simulink model "lab2_part3"  (R2023a)
settings: Solver=ode45  StartTime=0.0  StopTime=3  RelTol=1e-3
undefined symbols (not defined in the file or in its folder): a, zeta
settings Model: Creator=Jiadong_Hong  LastModifiedBy=Jiadong_Hong

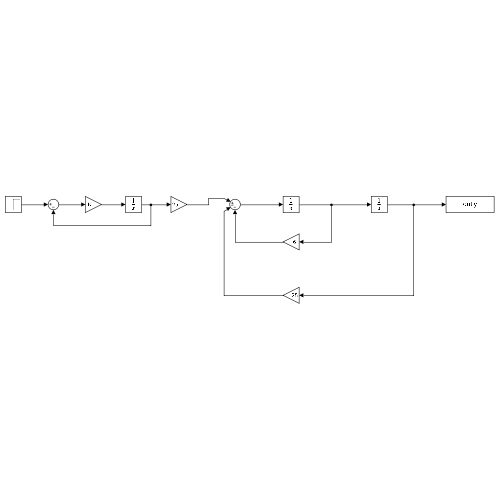
[thumbnail: Simulink's stored preview of the top-level diagram]
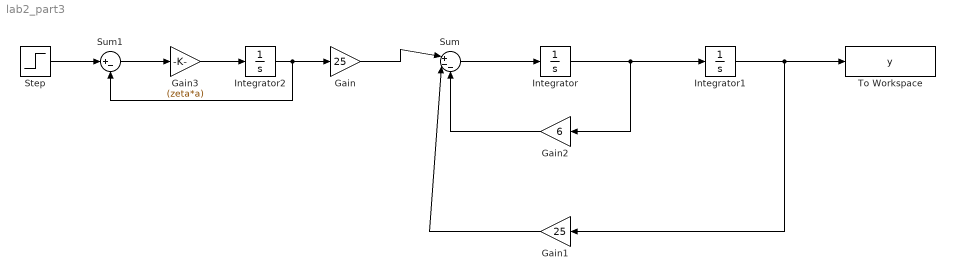
== system lab2_part3 ==
  Gain : Gain  Gain=25
  Gain1 : Gain  Gain=25
  Gain2 : Gain  Gain=6
  Gain3 : Gain  Gain=(zeta*a)
  Integrator : Integrator
  Integrator1 : Integrator
  Integrator2 : Integrator
  Step : Step  Time=0  SampleTime=0
  Sum : Sum  Inputs=|+--
  Sum1 : Sum  Inputs=|+-
  To Workspace : ToWorkspace  VariableName=y  SampleTime=-1
  wires:
  Gain/1 -> Sum/1
  Sum/1 -> Integrator/1
  Integrator1/1 -> Gain1/1, To Workspace/1
  Integrator/1 -> Integrator1/1, Gain2/1
  Gain1/1 -> Sum/2
  Gain2/1 -> Sum/3
  Step/1 -> Sum1/1
  Integrator2/1 -> Sum1/2, Gain/1
  Gain3/1 -> Integrator2/1
  Sum1/1 -> Gain3/1
